simulink model "MaglevNonLinear"  (R2018a)
settings: Solver=VariableStepAuto  StartTime=0.0  StopTime=10.0  RelTol=1e-3
settings Model: Creator=saad  LastModifiedBy=saad

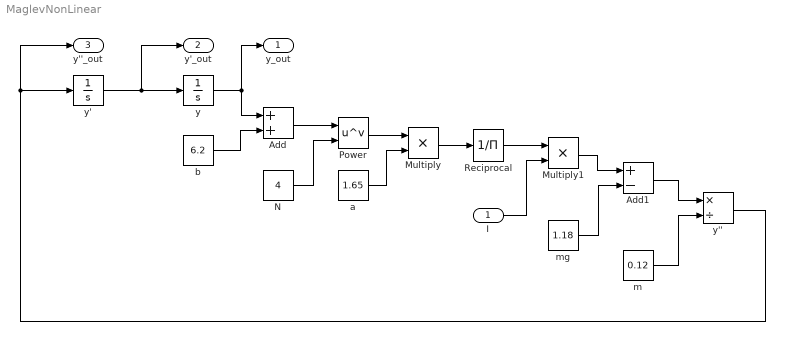
== system MaglevNonLinear ==
  I : Inport
  Add : Sum
  Add1 : Sum  Inputs=+-
  Multiply : Product
  Multiply1 : Product
  N : Constant  Value=4
  Power : Math  Operator=pow  SaturateOnIntegerOverflow=on
  Reciprocal : Product  Inputs=/
  a : Constant  Value=1.65
  b : Constant  Value=6.2
  m : Constant  Value=0.12
  mg : Constant  Value=1.18
  y : Integrator
  y' : Integrator
  y'' : Product  Inputs=*/
  y_out : Outport
  y'_out : Outport  Port=2
  y''_out : Outport  Port=3
  wires:
  y'/1 -> y'_out/1, y/1
  y/1 -> y_out/1, Add/1
  b/1 -> Add/2
  Add/1 -> Power/1
  N/1 -> Power/2
  Power/1 -> Multiply/1
  a/1 -> Multiply/2
  Multiply/1 -> Reciprocal/1
  Reciprocal/1 -> Multiply1/1
  I/1 -> Multiply1/2
  Multiply1/1 -> Add1/1
  mg/1 -> Add1/2
  Add1/1 -> y''/1
  m/1 -> y''/2
  y''/1 -> y''_out/1, y'/1
